simulink model "Target_Control_System"  (R2021b)
settings: Solver=FixedStepDiscrete  StartTime=0.0  StopTime=5  RelTol=1e-3
PreLoadFcn:
  | RTWConfigurationCB('preloadfcn', bdroot);
PostLoadFcn:
  | load('configuration/data_struct.mat');
  | load('configuration/fluxMaps_propMotor.mat');
  | load('configuration/parameterInit_PROP.mat');
  | load('configuration/parameterInit_PUMP.mat');
  | load('configuration/parameterInit_PITCH.mat');
  | load('configuration/parameterInit_TILT.mat');
  | %load('configuration/base_workspace_signal_definition.mat');
  | %load('resolvedatastores_to_baseworkspace_for_faster_simulation.mat');
model workspace (MAT data in the model file):
  SIMULATION_OPTIONS : Simulink.Parameter (value not decoded)
  TARGET_CODE_GEN : Simulink.Parameter (value not decoded)
  TCS_SAMPLE_FREQ_HZ : Simulink.Parameter (value not decoded)
symbols that are objects in the model workspace (value not decoded): TARGET_CODE_GEN, TCS_SAMPLE_FREQ_HZ
undefined symbols (not defined in the file): A_DQ_REF_LPF_INIT__PITCH, A_DQ_REF_LPF_INIT__PROP, A_DQ_REF_LPF_INIT__PUMP, A_DQ_REF_LPF_INIT__TILT, A_OBSERVER_CONFIDENCE_INIT__PITCH, A_OBSERVER_CONFIDENCE_INIT__PROP, A_OBSERVER_CONFIDENCE_INIT__PUMP, A_OBSERVER_CONFIDENCE_INIT__TILT, ACTUATOR_MAX_ANGLE_TRIP__PITCH, ACTUATOR_MIN_ANGLE_TRIP__PITCH, ACTUATOR_POS_SENSOR_INV_DIRECTION__PITCH, ACTUATOR_POS_SENSOR_INV_DIRECTION__TILT, ACTUATOR_POS_SENSOR_OFFSET__PITCH, ACTUATOR_POS_SENSOR_OFFSET__TILT, ADC_scaler1_baseaddr_TILT, ADC_SCALER_FLOAT_TO_FIXPOINT_EXPANSION, ANGLE_ELEC_FROM_SENSOR_OFFSET_INIT__PITCH, ANGLE_ELEC_FROM_SENSOR_OFFSET_INIT__PROP, ANGLE_ELEC_FROM_SENSOR_OFFSET_INIT__PUMP, ANGLE_ELEC_FROM_SENSOR_OFFSET_INIT__TILT, AUTO_CLEAR_FAULTS_ENABLED__PITCH, AUTO_CLEAR_FAULTS_ENABLED__PROP, AUTO_CLEAR_FAULTS_ENABLED__PUMP, AUTO_CLEAR_FAULTS_ENABLED__TILT, AUTO_CLEAR_FAULTS_WAIT_TICKS__PITCH, AUTO_CLEAR_FAULTS_WAIT_TICKS__PROP, AUTO_CLEAR_FAULTS_WAIT_TICKS__PUMP, AUTO_CLEAR_FAULTS_WAIT_TICKS__TILT, AUTO_I_ZERO_IDLE_TICKS__PITCH, AUTO_I_ZERO_IDLE_TICKS__PROP, AUTO_I_ZERO_IDLE_TICKS__PUMP, AUTO_I_ZERO_IDLE_TICKS__TILT, AUTO_I_ZERO_OFFSET_IDC_THRESHOLD__PITCH, AUTO_I_ZERO_OFFSET_IDC_THRESHOLD__PROP, AUTO_I_ZERO_OFFSET_IDC_THRESHOLD__PUMP, AUTO_I_ZERO_OFFSET_IDC_THRESHOLD__TILT, AUTO_I_ZERO_OFFSET_IPH_THRESHOLD__PITCH, AUTO_I_ZERO_OFFSET_IPH_THRESHOLD__PROP, AUTO_I_ZERO_OFFSET_IPH_THRESHOLD__PUMP, AUTO_I_ZERO_OFFSET_IPH_THRESHOLD__TILT, AUTO_SENSORLESS_SWITCHOVER_DISABLE_OMEGA, AUTO_SENSORLESS_SWITCHOVER_ENABLE_OMEGA, AUTO_SENSORLESS_SWITCHOVER_MIN_CONFIDENCE, AUXILIARY_PROTECTION_UNIT_BASEADDR__TILT, blanking_max_error_omega_INIT_PITCH, blanking_max_error_omega_INIT_TILT, blanking_max_error_position_INIT_PITCH, blanking_max_error_position_INIT_TILT, BRUTE_START_I_Q_REF_RAMP_SPEED__PITCH, BRUTE_START_I_Q_REF_RAMP_SPEED__PROP, BRUTE_START_I_Q_REF_RAMP_SPEED__PUMP, BRUTE_START_I_Q_REF_RAMP_SPEED__TILT, CONTROL_LOOP_DT_INIT__PITCH, CONTROL_LOOP_DT_INIT__PROP, CONTROL_LOOP_DT_INIT__PUMP, CONTROL_LOOP_DT_INIT__TILT, CORRECTION_FILTER_SCALE__PITCH, CORRECTION_FILTER_SCALE__PROP, CORRECTION_FILTER_SCALE__PUMP, CORRECTION_FILTER_SCALE__TILT ... (+458)
libraries: simulink x178, Reusables_Lib x24
(part 29 of 47)

== system Target_Control_System/Target_Control_System/MainLoop/pumpMotor_mainLoop/motorTaskMainFastStep(&oPump)/Control Loops - Pump/Dynamic Current Limiting Pump ==
  Enable : EnablePort
  Abs : Abs
  Add : Sum  Inputs=+-
  Add1 : Sum
  Add2 : Sum  Inputs=-+
  Data Store Read : DataStoreRead  DataStoreName=oPump  DataStoreElements=oPump.oMot_.oIn_.fIPhaseMagnitude_  IndexOptions=Index vector (dialog)  Indices=1  OutputSizes=1
  Data Store Read1 : DataStoreRead  DataStoreName=oPump  DataStoreElements=oPump.oMot_.oParam_.fIqSetpointMax_  IndexOptions=Index vector (dialog)  Indices=1  OutputSizes=1
  Data Store Read10 : DataStoreRead  DataStoreName=oPump  DataStoreElements=oPump.oMot_.oParam_.fDynILimIntegratorLeakageFactor_  IndexOptions=Index vector (dialog)  Indices=1  OutputSizes=1
  Data Store Read2 : DataStoreRead  DataStoreName=oPump  DataStoreElements=oPump.oMot_.oState_.fDynILimIntegrator_  IndexOptions=Index vector (dialog)  Indices=1  OutputSizes=1
  Data Store Read3 : DataStoreRead  DataStoreName=oPump  DataStoreElements=oPump.oMot_.oParam_.fDynILimDynamicMax_  IndexOptions=Index vector (dialog)  Indices=1  OutputSizes=1
  Data Store Read4 : DataStoreRead  DataStoreName=oPump  DataStoreElements=oPump.oMot_.oParam_.fTorqueAuthorityFraction_  IndexOptions=Index vector (dialog)  Indices=1  OutputSizes=1
  Data Store Read5 : DataStoreRead  DataStoreName=oPump  DataStoreElements=oPump.oMot_.oParam_.fDynILimKnockdownFactor_  IndexOptions=Index vector (dialog)  Indices=1  OutputSizes=1
  Data Store Read6 : DataStoreRead  DataStoreName=oPump  DataStoreElements=oPump.oMot_.oState_.fIqRefBeforeRamp_  IndexOptions=Index vector (dialog)  Indices=1  OutputSizes=1
  Data Store Read7 : DataStoreRead  DataStoreName=oPump  DataStoreElements=oPump.oMot_.oParam_.fDynILimDynamicMax_  IndexOptions=Index vector (dialog)  Indices=1  OutputSizes=1
  Data Store Write : DataStoreWrite  DataStoreName=oPump  DataStoreElements=oPump.oMot_.oState_.fDynILimIntegrator_  IndexOptions=Index vector (dialog)  Indices=1  OutputSizes=1
  Data Store Write1 : DataStoreWrite  DataStoreName=oPump  DataStoreElements=oPump.oMot_.oState_.fDynILimActualLimit_  IndexOptions=Index vector (dialog)  Indices=1  OutputSizes=1
  Data Store Write3 : DataStoreWrite  DataStoreName=oPump  DataStoreElements=oPump.oMot_.oParam_.oPid2DataRpmCtrl_.oParameter_.fOutMax_  IndexOptions=Index vector (dialog)  Indices=1  OutputSizes=1
  Data Store Write4 : DataStoreWrite  DataStoreName=oPump  DataStoreElements=oPump.oMot_.oParam_.oPid2DataRpmCtrl_.oParameter_.fOutMin_  IndexOptions=Index vector (dialog)  Indices=1  OutputSizes=1
  Data Store Write5 : DataStoreWrite  DataStoreName=oPump  DataStoreElements=oPump.oMot_.oParam_.oPid2DataRpmCtrl_.oParameter_.fIntMin_  IndexOptions=Index vector (dialog)  Indices=1  OutputSizes=1
  Data Store Write6 : DataStoreWrite  DataStoreName=oPump  DataStoreElements=oPump.oMot_.oParam_.oPid2DataRpmCtrl_.oParameter_.fIntMax_  IndexOptions=Index vector (dialog)  Indices=1  OutputSizes=1
  Divide{,1..3} (4 alike) : Product  Inputs=**
  Gain : Gain  Gain=-1
  Gain1 : Gain  Gain=-1
  Gain2 : Gain  Gain=-1
  Max : MinMax  Function=max  Inputs=2
  Max1 : MinMax  Function=max  Inputs=2
  Min : MinMax  Inputs=2
  Switch : Switch  Criteria=u2 > Threshold
  oRampDataIqRef_.fSetpoint : Outport
  wires:
  Gain2/1 -> Data Store Write4/1
  Data Store Read7/1 -> Gain2/1, Data Store Write3/1
  Gain1/1 -> Data Store Write5/1
  Max1/1 -> oRampDataIqRef_.fSetpoint/1
  Gain/1 -> Max1/1
  Min/1 -> Max1/2
  Data Store Read6/1 -> Min/2
  Max/1 -> Min/1, Data Store Write1/1, Gain1/1, Data Store Write6/1, Gain/1
  Add2/1 -> Max/1
  Divide2/1 -> Add2/2
  Divide3/1 -> Add2/1
  Data Store Read5/1 -> Divide3/2
  Data Store Read4/1 -> Divide2/2
  Data Store Read3/1 -> Divide2/1
  Divide1/1 -> Switch/3
  Data Store Read10/1 -> Divide1/2
  Data Store Read2/1 -> Add1/2, Divide1/1
  Divide/1 -> Add1/1
  Switch/1 -> Divide3/1, Data Store Write/1
  Add1/1 -> Switch/1
  Add/1 -> Switch/2, Divide/2, Divide/1  "fTemp"
  Abs/1 -> Add/1
  Data Store Read1/1 -> Add/2, Max/2
  Data Store Read/1 -> Abs/1

== system Target_Control_System/Target_Control_System/MainLoop/pumpMotor_mainLoop/motorTaskMainFastStep(&oPump)/Control Loops - Pump/Sim Options Prop Id Variant Subsystem ==
  note: 1) Add Subsystem or Model blocks as valid variant choices.
      | 2) You cannot connect blocks at this level. At simulation, connectivity is automatically
      | determined, based on the active variant and port name matching.
  Sim Options 0 Prop Id Subsystem : Subsystem  VariantControl=(default)
  Sim Options 1 Prop Id Subsystem : Subsystem  VariantControl=SIMULATION_OPTIONS == 1 && TARGET_CODE_GEN ~= 1
  Out1 : Outport

== system Target_Control_System/Target_Control_System/MainLoop/pumpMotor_mainLoop/motorTaskMainFastStep(&oPump)/Control Loops - Pump/Sim Options Pump Iq Variant Subsystem ==
  note: 1) Add Subsystem or Model blocks as valid variant choices.
      | 2) You cannot connect blocks at this level. At simulation, connectivity is automatically
      | determined, based on the active variant and port name matching.
  Sim Options 0 Pump Iq Subsystem : Subsystem  VariantControl=(default)
  Sim Options 1 Pump Iq Subsystem : Subsystem  VariantControl=SIMULATION_OPTIONS == 1 && TARGET_CODE_GEN ~= 1
  fSetpoint_ : Outport

== system Target_Control_System/Target_Control_System/MainLoop/pumpMotor_mainLoop/motorTaskMainFastStep(&oPump)/Control Loops - Pump/Sim Options Pump OmegaERef Variant Subsystem ==
  note: 1) Add Subsystem or Model blocks as valid variant choices.
      | 2) You cannot connect blocks at this level. At simulation, connectivity is automatically
      | determined, based on the active variant and port name matching.
  Sim Options 0 Pump OmegaE Subsystem : Subsystem  VariantControl=(default)
  Sim Options 1 Pump OmegaE Subsystem : Subsystem  VariantControl=SIMULATION_OPTIONS == 1 && TARGET_CODE_GEN ~= 1
  Out1 : Outport

== system Target_Control_System/Target_Control_System/MainLoop/pumpMotor_mainLoop/motorTaskMainFastStep(&oPump)/Control Loops - Pump/Subsystem ==
  note: // Drives without sensors use the PI type controller and the estimated speed
  note: // Drives with sensors use the PID2 controller and the sensor (derived or reported) speed
  note: // Drive states 245-255 are for resistance measurement
  In Bus Element : Inport  PortName=oRampDataOmegaERef_.fRampOut
  In Bus Element1 : Inport  PortName=oRampDataOmegaERef_.fRampOut
  Enable : EnablePort
  AND : Logic  AllPortsSameDT=off  OutDataTypeStr=boolean
  Constant : Constant  OutDataTypeStr=single  SampleTime=-1
  Constant1 : Constant  OutDataTypeStr=single  SampleTime=-1
  Constant2 : Constant  Value=245  OutDataTypeStr=uint32  SampleTime=-1
  Data Store Read2 : DataStoreRead  DataStoreName=oPump  DataStoreElements=oPump.oMot_.oIn_.fOmegaEObserverLpf2_  IndexOptions=Index vector (dialog)  Indices=1  OutputSizes=1
  Data Store Read4 : DataStoreRead  DataStoreName=oPump  DataStoreElements=oPump.oMot_.oParam_.oPid2DataRpmCtrl_.fState_  IndexOptions=Index vector (dialog)  Indices=1  OutputSizes=1
  Data Store Read5 : DataStoreRead  DataStoreName=oPump  DataStoreElements=oPump.oMot_.oParam_.uiTorqueMirroringActive_  IndexOptions=Index vector (dialog)  Indices=1  OutputSizes=1
  Data Store Read6 : DataStoreRead  DataStoreName=oPump  DataStoreElements=oPump.oMot_.oState_.uiDriveState_  IndexOptions=Index vector (dialog)  Indices=1  OutputSizes=1
  Data Store Read62 : DataStoreRead  DataStoreName=oPump  DataStoreElements=oPump.oIsr_.oParam_.iUseSensorAngle_  IndexOptions=Index vector (dialog)  Indices=1  OutputSizes=1
  Data Store Read7 : DataStoreRead  DataStoreName=oPump  DataStoreElements=oPump.oMot_.oState_.oPosSensor_.fOmegaEFromSensor_  IndexOptions=Index vector (dialog)  Indices=1  OutputSizes=1
  Data Store Write19 : DataStoreWrite  DataStoreName=oPump  DataStoreElements=oPump.oMot_.oState_.fIqRefBeforeRamp_  IndexOptions=Index vector (dialog)  Indices=1  OutputSizes=1
  Data Store Write5 : DataStoreWrite  DataStoreName=oPump  DataStoreElements=oPump.oMot_.oState_.fIqRefFromSpeedController_  IndexOptions=Index vector (dialog)  Indices=1  OutputSizes=1
  Less Than : RelationalOperator  Operator=<  OutDataTypeStr=boolean  RndMeth=Simplest
  NOT : Logic  Operator=NOT  AllPortsSameDT=off  OutDataTypeStr=boolean
  NOT1 : Logic  Operator=NOT  AllPortsSameDT=off  OutDataTypeStr=boolean
  Set Iq Ref Pump : Subsystem  TreatAsAtomicUnit=on
  Switch : Switch  Criteria=u2 > Threshold
  piControllerStep(&oPiDataRpm_) : Subsystem
  pid2ControllerStep(&oPid2DataRpmCtrl_) : Subsystem
  wires:
  Set Iq Ref Pump/1(fIqRefBeforeRamp) -> Data Store Write19/1
  AND/1 -> Set Iq Ref Pump/Enable
  Less Than/1 -> AND/2
  NOT1/1 -> AND/1
  Data Store Read5/1 -> NOT1/1
  Data Store Read6/1 -> Less Than/1
  Constant2/1 -> Less Than/2
  Switch/1 -> Data Store Write5/1, Set Iq Ref Pump/1(fIqRefFromSpeedController)
  pid2ControllerStep(&oPid2DataRpmCtrl_)/1(fOutput) -> Switch/1
  Data Store Read7/1 -> pid2ControllerStep(&oPid2DataRpmCtrl_)/2(fActual)
  Data Store Read4/1 -> pid2ControllerStep(&oPid2DataRpmCtrl_)/1(fState)
  Constant1/1 -> pid2ControllerStep(&oPid2DataRpmCtrl_)/4(fActualDdt)
  In Bus Element/1 -> pid2ControllerStep(&oPid2DataRpmCtrl_)/3(fTarget)
  Data Store Read2/1 -> piControllerStep(&oPiDataRpm_)/1(fActual)
  piControllerStep(&oPiDataRpm_)/1(fOutput) -> Switch/3
  In Bus Element1/1 -> piControllerStep(&oPiDataRpm_)/2(fTarget)
  Constant/1 -> piControllerStep(&oPiDataRpm_)/3(fScale)
  Data Store Read62/1 -> Switch/2, pid2ControllerStep(&oPid2DataRpmCtrl_)/Enable, NOT/1
  NOT/1 -> piControllerStep(&oPiDataRpm_)/Enable

== system Target_Control_System/Target_Control_System/MainLoop/pumpMotor_mainLoop/motorTaskMainFastStep(&oPump)/Control Loops - Pump/Subsystem2 ==
  Enable : EnablePort
  Data Store Read2 : DataStoreRead  DataStoreName=oPump  DataStoreElements=oPump.oMot_.oIn_.fUdRef_  IndexOptions=Index vector (dialog)  Indices=1  OutputSizes=1
  Data Store Read3 : DataStoreRead  DataStoreName=oPump  DataStoreElements=oPump.oMot_.oIn_.fUqRef_  IndexOptions=Index vector (dialog)  Indices=1  OutputSizes=1
  Data Store Read5 : DataStoreRead  DataStoreName=oPump  DataStoreElements=oPump.oMot_.oState_.fFluxWeakeningState_  IndexOptions=Index vector (dialog)  Indices=1  OutputSizes=1
  Data Store Read6 : DataStoreRead  DataStoreName=oPump  DataStoreElements=oPump.oMot_.oParam_.fFluxWeakeningModulationTarget_  IndexOptions=Index vector (dialog)  Indices=1  OutputSizes=1
  Data Store Read69 : DataStoreRead  DataStoreName=oPump  DataStoreElements=oPump.oMot_.oParam_.fFluxWeakeningDownRamp_  IndexOptions=Index vector (dialog)  Indices=1  OutputSizes=1
  Data Store Read94 : DataStoreRead  DataStoreName=oPump  DataStoreElements=oPump.oMot_.oState_.fFluxWeakeningState_  IndexOptions=Index vector (dialog)  Indices=1  OutputSizes=1
  Data Store Read95 : DataStoreRead  DataStoreName=oPump  DataStoreElements=oPump.oMot_.oParam_.fIntControlLoopDt_  IndexOptions=Index vector (dialog)  Indices=1  OutputSizes=1
  Data Store Read96 : DataStoreRead  DataStoreName=oPump  DataStoreElements=oPump.oMot_.oParam_.fIntControlLoopDt_  IndexOptions=Index vector (dialog)  Indices=1  OutputSizes=1
  Equal13 : RelationalOperator  Operator=<  OutDataTypeStr=boolean  RndMeth=Simplest
  Mux : Mux  Inputs=2
  NOT1 : Logic  Operator=NOT  AllPortsSameDT=off  OutDataTypeStr=boolean
  Square Sum : Fcn  Expr=u(1)*u(1)+u(2)*u(2)
  Subsystem : Subsystem
  Subsystem1 : Subsystem
  Switch1 : Switch  Criteria=u2 > Threshold  Threshold=0.5
  Out1 : Outport
  wires:
  Subsystem1/1(Out1) -> Switch1/1
  NOT1/1 -> Subsystem/Enable
  Data Store Read94/1 -> Subsystem/3(fFluxWeakeningState_)
  Subsystem/1(Out1) -> Switch1/3
  Mux/1 -> Square Sum/1
  Data Store Read95/1 -> Subsystem/4(fIntControlLoopDt_)
  Data Store Read6/1 -> Equal13/2, Subsystem/1(fFluxWeakeningModulationTarget_)  "fFluxWeakeningModulationTarget_"
  Square Sum/1 -> Subsystem/2(fModulationIndexSquared), Equal13/1  "fModulationIndexSquared_"
  Data Store Read3/1 -> Mux/2
  Equal13/1 -> Subsystem1/Enable, NOT1/1, Switch1/2
  Data Store Read96/1 -> Subsystem1/2(fIntControlLoopDt_)
  Switch1/1 -> Out1/1
  Data Store Read2/1 -> Mux/1
  Data Store Read69/1 -> Subsystem1/1(fFluxWeakeningDownRamp_)
  Data Store Read5/1 -> Subsystem1/3(fFluxWeakeningState_)

== system Target_Control_System/Target_Control_System/MainLoop/pumpMotor_mainLoop/motorTaskMainFastStep(&oPump)/Control Loops - Pump/rampStep_oRampDataIqRef_ ==
  note: U(k)
  note: Y(k)
  fSetpoint_ : Inport
  fUpslope_ : Inport  Port=2
  fDDownslope_ : Inport  Port=3
  fTimestepS_ : Inport  Port=4
  fRampOut_z : Inport  Port=5
  Difference Inputs1 : Sum  Description=Add in CPU  DisableCoverage=on  Inputs=+-  OutDataTypeStr=Inherit: Inherit via back propagation
  Difference Inputs2 : Sum  Description=Add in CPU  OutDataTypeStr=Inherit: Inherit via back propagation
  Difference Inputs3 : Sum  Description=Add in CPU  DisableCoverage=on  Inputs=+-  OutDataTypeStr=Inherit: Inherit via back propagation
  Gain : Gain  Gain=-1
  Saturation Dynamic : simulink/Discontinuities/Saturation Dynamic  OutMin=[]  OutMax=[]  OutDataTypeStr=Inherit: Same as second input  OutDataType=fixdt(1, 16)  OutScaling=2^-10  DoSatur=off
  delta fall limit : Product  DisableCoverage=on  Inputs=**  OutDataTypeStr=Inherit: Inherit via back propagation  SaturateOnIntegerOverflow=on
  delta fall limit1 : Product  DisableCoverage=on  Inputs=*/  OutDataTypeStr=Inherit: Inherit via back propagation  SaturateOnIntegerOverflow=on
  delta rise limit : Product  DisableCoverage=on  Inputs=**  OutDataTypeStr=Inherit: Inherit via back propagation  SaturateOnIntegerOverflow=on
  fRampOut_ : Outport  InitialOutput=0
  fRampOutDdt_ : Outport  Port=2  InitialOutput=0
  wires:
  fRampOut_z/1 -> Difference Inputs1/2, Difference Inputs2/2, Difference Inputs3/2
  Difference Inputs1/1 -> Saturation Dynamic/2  "( U(k) - Y(k-1) )"
  fDDownslope_/1 -> Gain/1
  delta rise limit/1 -> Saturation Dynamic/1
  fSetpoint_/1 -> Difference Inputs1/1
  delta fall limit/1 -> Saturation Dynamic/3
  fUpslope_/1 -> delta rise limit/1
  Difference Inputs2/1 -> Difference Inputs3/1, fRampOut_/1
  Saturation Dynamic/1 -> Difference Inputs2/1
  fTimestepS_/1 -> delta fall limit1/2, delta fall limit/2, delta rise limit/2
  Difference Inputs3/1 -> delta fall limit1/1  "( Y(k) - Y(k-1) )"
  delta fall limit1/1 -> fRampOutDdt_/1
  Gain/1 -> delta fall limit/1

== system Target_Control_System/Target_Control_System/MainLoop/pumpMotor_mainLoop/motorTaskMainFastStep(&oPump)/Correction Constants for Observer and Control - Pump/Variant Subsystem ==
  note: 1) Add Subsystem or Model blocks as valid variant choices.
      | 2) You cannot connect blocks at this level. At simulation, connectivity is automatically
      | determined, based on the active variant and port name matching.
  In1 : Inport
  Simulation Subsystem IIR Voltage Filter Freq : Subsystem  TreatAsAtomicUnit=on  VariantControl=TARGET_CODE_GEN == 0
  Target Code Gen Subsystem IIR Voltage Filter Freq : Subsystem  TreatAsAtomicUnit=on  VariantControl="TARGET_CODE_GEN  == 1"
  Out1 : Outport

== system Target_Control_System/Target_Control_System/MainLoop/pumpMotor_mainLoop/motorTaskMainFastStep(&oPump)/Observer Confidence - Pump/IIR ==
  In : Inport
  1-K : Inport  Port=2
  K : Inport  Port=3
  Product : Product  OutDataTypeStr=single  RndMeth=Zero
  Product1 : Product  RndMeth=Zero
  Sum : Sum  Inputs=|++  OutDataTypeStr=single
  Unit Delay : UnitDelay  SampleTime=-1  HasFrameUpgradeWarning=on
  Out : Outport
  wires:
  Sum/1 -> Unit Delay/1, Out/1
  Unit Delay/1 -> Product/1
  K/1 -> Product1/2
  1-K/1 -> Product/2
  Product/1 -> Sum/1
  Product1/1 -> Sum/2
  In/1 -> Product1/1

== system Target_Control_System/Target_Control_System/MainLoop/pumpMotor_mainLoop/motorTaskMainFastStep(&oPump)/PWM for Simulation/Subsystem ==
  Enable : EnablePort
  Bus Creator1 : BusCreator  Inputs=3
  Data Store Read7 : DataStoreRead  DataStoreName=oPump  DataStoreElements=oPump.oIsr_.oOut_.uiPwmDutyTicksA_  IndexOptions=Index vector (dialog)  Indices=1  OutputSizes=1
  Data Store Read8 : DataStoreRead  DataStoreName=oPump  DataStoreElements=oPump.oIsr_.oOut_.uiPwmDutyTicksB_  IndexOptions=Index vector (dialog)  Indices=1  OutputSizes=1
  Data Store Read9 : DataStoreRead  DataStoreName=oPump  DataStoreElements=oPump.oIsr_.oOut_.uiPwmDutyTicksC_  IndexOptions=Index vector (dialog)  Indices=1  OutputSizes=1
  pumpMotor_PWMticks : Outport
  wires:
  Data Store Read8/1 -> Bus Creator1/2  "Bticks"
  Bus Creator1/1 -> pumpMotor_PWMticks/1
  Data Store Read9/1 -> Bus Creator1/3  "Cticks"
  Data Store Read7/1 -> Bus Creator1/1  "Aticks"

== system Target_Control_System/Target_Control_System/MainLoop/pumpMotor_mainLoop/motorTaskMainFastStep(&oPump)/PWM for Simulation/Subsystem1 ==
  Enable : EnablePort
  Data Store Read6 : DataStoreRead  DataStoreName=oPump  DataStoreElements=oPump.oMot_.oOut_.uiPwmRequestFromMain_  IndexOptions=Index vector (dialog)  Indices=1  OutputSizes=1
  Scope : Scope
  Subsystem : Subsystem
  pumpMotor_PWMticks : Outport
  wires:
  Data Store Read6/1 -> Subsystem/Enable, Scope/1
  Subsystem/1(pumpMotor_PWMticks) -> pumpMotor_PWMticks/1

== system Target_Control_System/Target_Control_System/MainLoop/pumpMotor_mainLoop/motorTaskMainFastStep(&oPump)/Variant Subsystem/Target_Code_Gen_0 ==
  Function-Call Generator : simulink/Ports & Subsystems/Function-Call Generator  sample_time=-1  numberOfIterations=1  DisallowWideOutput=off
  Output : Outport
  wires:
  Function-Call Generator/1 -> Output/1

== system Target_Control_System/Target_Control_System/MainLoop/pumpMotor_mainLoop/motorTaskMainFastStep(&oPump)/Variant Subsystem/Target_Code_Gen_1 ==
  Data Store Read16 : DataStoreRead  DataStoreName=oPump  DataStoreElements=oPump.oMot_.oIn_.uiDataFromIsrToMainUpdated_  IndexOptions=Index vector (dialog)  Indices=1  OutputSizes=1
  Triggered Subsystem : Subsystem  TreatAsAtomicUnit=on
  Output : Outport
  wires:
  Triggered Subsystem/1(Output) -> Output/1
  Data Store Read16/1 -> Triggered Subsystem/Trigger

== system Target_Control_System/Target_Control_System/MainLoop/tiltMotor_mainLoop/Decimation gate for 10 Hz Tilt/Function-Call Subsystem/Dynamic_current_limiting ==
  Constant : Constant  Value=0  OutDataTypeStr=single  SampleTime=-1
  Data Store Read2 : DataStoreRead  DataStoreName=oTilt  DataStoreElements=oTilt.oMot_.oParam_.fDynILimIntegratorLeakageFactor_  IndexOptions=Index vector (dialog)  Indices=1  OutputSizes=1
  Enabled Subsystem : Subsystem  TreatAsAtomicUnit=on
  GreaterThan : RelationalOperator  Operator=>  OutDataTypeStr=boolean  RndMeth=Simplest
  wires:
  GreaterThan/1 -> Enabled Subsystem/Enable
  Data Store Read2/1 -> GreaterThan/1
  Constant/1 -> GreaterThan/2

== system Target_Control_System/Target_Control_System/MainLoop/tiltMotor_mainLoop/Decimation gate for 200 Hz Tilt/motorTaskMainDecimationAStep(&oTilt)/Check zero current if inverter off ==
  function : TriggerPort  TriggerType=function-call  VariantControl=Variant
  AND : Logic  Inputs=3  AllPortsSameDT=off  OutDataTypeStr=boolean
  Constant : Constant  Value=200  OutDataTypeStr=uint32  SampleTime=-1
  Constant1 : Constant  Value=99  OutDataTypeStr=uint32  SampleTime=-1
  Constant2 : Constant  Value=0  OutDataTypeStr=uint32  SampleTime=-1
  Data Store Read1 : DataStoreRead  DataStoreName=oTilt  DataStoreElements=oTilt.oMot_.oState_.uiDriveState_  IndexOptions=Index vector (dialog)  Indices=1  OutputSizes=1
  Data Store Read2 : DataStoreRead  DataStoreName=oTilt  DataStoreElements=oTilt.oMot_.oState_.uiCurrentOffsetNullingPerformed_  IndexOptions=Index vector (dialog)  Indices=1  OutputSizes=1
  Enabled Subsystem : Subsystem  TreatAsAtomicUnit=on
  GreaterThan : RelationalOperator  Operator=>  OutDataTypeStr=boolean  RndMeth=Simplest
  GreaterThan1 : RelationalOperator  Operator=>  OutDataTypeStr=boolean  RndMeth=Simplest
  Less Than : RelationalOperator  Operator=<  OutDataTypeStr=boolean  RndMeth=Simplest
  wires:
  AND/1 -> Enabled Subsystem/Enable
  GreaterThan1/1 -> AND/3
  Constant2/1 -> GreaterThan1/2
  Data Store Read2/1 -> GreaterThan1/1
  Less Than/1 -> AND/2
  GreaterThan/1 -> AND/1
  Constant1/1 -> GreaterThan/2
  Constant/1 -> Less Than/2
  Data Store Read1/1 -> GreaterThan/1, Less Than/1

== system Target_Control_System/Target_Control_System/MainLoop/tiltMotor_mainLoop/Decimation gate for 200 Hz Tilt/motorTaskMainDecimationAStep(&oTilt)/Current control inactive ==
  function : TriggerPort  TriggerType=function-call  VariantControl=Variant
  Constant : Constant  Value=0  OutDataTypeStr=uint32  SampleTime=-1
  Data Store Read : DataStoreRead  DataStoreName=oTilt  DataStoreElements=oTilt.oMot_.oOut_.uiCurrentControllerActive_  IndexOptions=Index vector (dialog)  Indices=1  OutputSizes=1
  Enabled Subsystem : Subsystem  TreatAsAtomicUnit=on
  GreaterThan : RelationalOperator  Operator=>  OutDataTypeStr=boolean  RndMeth=Simplest
  NOT : Logic  Operator=NOT  IconShape=distinctive  AllPortsSameDT=off  OutDataTypeStr=boolean
  wires:
  NOT/1 -> Enabled Subsystem/Enable
  GreaterThan/1 -> NOT/1
  Constant/1 -> GreaterThan/2
  Data Store Read/1 -> GreaterThan/1

== system Target_Control_System/Target_Control_System/MainLoop/tiltMotor_mainLoop/Decimation gate for 200 Hz Tilt/motorTaskMainDecimationAStep(&oTilt)/Current offset nulling ==
  note: Try to perform current sensor offset nulling at least once as soon as possible:
      | (Subsequent nulling steps are performed only once the drive has been idle for a while)
  function : TriggerPort  TriggerType=function-call  VariantControl=Variant
  Constant2 : Constant  Value=0  OutDataTypeStr=uint32  SampleTime=-1
  Data Store Read2 : DataStoreRead  DataStoreName=oTilt  DataStoreElements=oTilt.oMot_.oState_.uiCurrentOffsetNullingPerformed_  IndexOptions=Index vector (dialog)  Indices=1  OutputSizes=1
  GreaterThan1 : RelationalOperator  Operator=>  OutDataTypeStr=boolean  RndMeth=Simplest
  NOT : Logic  Operator=NOT  IconShape=distinctive  AllPortsSameDT=off  OutDataTypeStr=boolean
  initiateOffsetNulling(&oTilt) : Subsystem  TreatAsAtomicUnit=on
  wires:
  NOT/1 -> initiateOffsetNulling(&oTilt)/Enable
  GreaterThan1/1 -> NOT/1
  Constant2/1 -> GreaterThan1/2
  Data Store Read2/1 -> GreaterThan1/1

== system Target_Control_System/Target_Control_System/MainLoop/tiltMotor_mainLoop/Decimation gate for 200 Hz Tilt/motorTaskMainDecimationAStep(&oTilt)/DClink_overCurrentProtection ==
  function : TriggerPort  TriggerType=function-call  VariantControl=Variant
  Chart : Stateflow chart  TreatAsAtomicUnit=on

== system Target_Control_System/Target_Control_System/MainLoop/tiltMotor_mainLoop/Decimation gate for 200 Hz Tilt/motorTaskMainDecimationAStep(&oTilt)/Forced current injection for broken input sensors ==
  function : TriggerPort  TriggerType=function-call  VariantControl=Variant
  Constant : Constant  Value=226  OutDataTypeStr=uint32  SampleTime=-1
  Constant1 : Constant  Value=227  OutDataTypeStr=uint32  SampleTime=-1
  Constant2 : Constant  Value=228  OutDataTypeStr=uint32  SampleTime=-1
  Data Store Read : DataStoreRead  DataStoreName=oTilt  DataStoreElements=oTilt.oMot_.oState_.uiDriveState_  IndexOptions=Index vector (dialog)  Indices=1  OutputSizes=1
  Enabled Subsystem : Subsystem  TreatAsAtomicUnit=on
  Equal : RelationalOperator  Operator===  OutDataTypeStr=boolean  RndMeth=Simplest
  Equal1 : RelationalOperator  Operator===  OutDataTypeStr=boolean  RndMeth=Simplest
  Equal2 : RelationalOperator  Operator===  OutDataTypeStr=boolean  RndMeth=Simplest
  OR : Logic  Operator=OR  Inputs=3  AllPortsSameDT=off  OutDataTypeStr=boolean
  wires:
  OR/1 -> Enabled Subsystem/Enable
  Equal2/1 -> OR/3
  Equal/1 -> OR/1
  Equal1/1 -> OR/2
  Constant2/1 -> Equal2/2
  Constant1/1 -> Equal1/2
  Constant/1 -> Equal/2
  Data Store Read/1 -> Equal/1, Equal1/1, Equal2/1

== system Target_Control_System/Target_Control_System/MainLoop/tiltMotor_mainLoop/Decimation gate for 200 Hz Tilt/motorTaskMainDecimationAStep(&oTilt)/Idle controller ==
  function : TriggerPort  TriggerType=function-call  VariantControl=Variant
  Constant : Constant  Value=211  OutDataTypeStr=uint32  SampleTime=-1
  Constant1 : Constant  Value=212  OutDataTypeStr=uint32  SampleTime=-1
  Data Store Read : DataStoreRead  DataStoreName=oTilt  DataStoreElements=oTilt.oMot_.oState_.uiDriveState_  IndexOptions=Index vector (dialog)  Indices=1  OutputSizes=1
  Equal : RelationalOperator  Operator===  OutDataTypeStr=boolean  RndMeth=Simplest
  Equal1 : RelationalOperator  Operator===  OutDataTypeStr=boolean  RndMeth=Simplest
  Forced angle : Subsystem  TreatAsAtomicUnit=on
  NOT : Logic  Operator=NOT  IconShape=distinctive  AllPortsSameDT=off  OutDataTypeStr=boolean
  Not forced angle : Subsystem  TreatAsAtomicUnit=on
  OR : Logic  Operator=OR  AllPortsSameDT=off  OutDataTypeStr=boolean
  wires:
  NOT/1 -> Not forced angle/Enable
  OR/1 -> NOT/1, Forced angle/Enable
  Equal1/1 -> OR/2
  Equal/1 -> OR/1
  Constant1/1 -> Equal1/2
  Data Store Read/1 -> Equal/1, Equal1/1
  Constant/1 -> Equal/2

== system Target_Control_System/Target_Control_System/MainLoop/tiltMotor_mainLoop/Decimation gate for 200 Hz Tilt/motorTaskMainDecimationAStep(&oTilt)/Position control checks ==
  function : TriggerPort  TriggerType=function-call  VariantControl=Variant
  Constant : Constant  Value=0  OutDataTypeStr=int32  SampleTime=-1
  Data Store Read : DataStoreRead  DataStoreName=oTilt  DataStoreElements=oTilt.oMot_.oState_.oPosSensor_.iPosControlEnabled_  IndexOptions=Index vector (dialog)  Indices=1  OutputSizes=1
  GreaterThan : RelationalOperator  Operator=>  OutDataTypeStr=boolean  RndMeth=Simplest
  NOT : Logic  Operator=NOT  IconShape=distinctive  AllPortsSameDT=off  OutDataTypeStr=boolean
  NOT position control mode : Subsystem  TreatAsAtomicUnit=on
  Position control mode : Subsystem  TreatAsAtomicUnit=on
  wires:
  NOT/1 -> NOT position control mode/Enable
  Constant/1 -> GreaterThan/2
  Data Store Read/1 -> GreaterThan/1
  GreaterThan/1 -> Position control mode/Enable, NOT/1

== system Target_Control_System/Target_Control_System/MainLoop/tiltMotor_mainLoop/Decimation gate for 5000 Hz Tilt/motorTaskProcessExternalSetpoints(&oTilt)/hot_standby ==
  hot_standby : TriggerPort  TriggerType=function-call  VariantControl=Variant
  AND5 : Logic  Operator=OR  AllPortsSameDT=off  OutDataTypeStr=boolean
  Data Store Read85 : DataStoreRead  DataStoreName=oTilt  DataStoreElements=oTilt.oMot_.oState_.uiDriveState_  IndexOptions=Index vector (dialog)  Indices=1  OutputSizes=1
  Equal1 : RelationalOperator  Operator===  OutDataTypeStr=boolean  RndMeth=Simplest
  Equal13 : RelationalOperator  Operator===  OutDataTypeStr=boolean  RndMeth=Simplest
  Subsystem : Subsystem
  const1 : Constant  Value=235  OutDataTypeStr=uint32  SampleTime=-1
  const2 : Constant  Value=236  OutDataTypeStr=uint32  SampleTime=-1
  wires:
  const2/1 -> Equal1/2
  const1/1 -> Equal13/2
  Data Store Read85/1 -> Equal13/1, Equal1/1
  Equal1/1 -> AND5/2
  AND5/1 -> Subsystem/Enable
  Equal13/1 -> AND5/1

== system Target_Control_System/Target_Control_System/MainLoop/tiltMotor_mainLoop/Decimation gate for 5000 Hz Tilt/motorTaskProcessExternalSetpoints(&oTilt)/passive_holding_mode ==
  passive_holding_mode : TriggerPort  TriggerType=function-call  VariantControl=Variant
  AND5 : Logic  Operator=OR  Inputs=3  AllPortsSameDT=off  OutDataTypeStr=boolean
  Data Store Read85 : DataStoreRead  DataStoreName=oTilt  DataStoreElements=oTilt.oMot_.oState_.uiDriveState_  IndexOptions=Index vector (dialog)  Indices=1  OutputSizes=1
  Equal1 : RelationalOperator  Operator===  OutDataTypeStr=boolean  RndMeth=Simplest
  Equal13 : RelationalOperator  Operator===  OutDataTypeStr=boolean  RndMeth=Simplest
  Equal2 : RelationalOperator  Operator===  OutDataTypeStr=boolean  RndMeth=Simplest
  Subsystem : Subsystem
  const1 : Constant  Value=226  OutDataTypeStr=uint32  SampleTime=-1
  const2 : Constant  Value=227  OutDataTypeStr=uint32  SampleTime=-1
  const3 : Constant  Value=228  OutDataTypeStr=uint32  SampleTime=-1
  wires:
  const3/1 -> Equal2/2
  const2/1 -> Equal1/2
  const1/1 -> Equal13/2
  Data Store Read85/1 -> Equal13/1, Equal1/1, Equal2/1
  Equal1/1 -> AND5/2
  Equal2/1 -> AND5/3
  AND5/1 -> Subsystem/Enable
  Equal13/1 -> AND5/1

== system Target_Control_System/Target_Control_System/MainLoop/tiltMotor_mainLoop/Decimation gate for 5000 Hz Tilt/motorTaskProcessExternalSetpoints(&oTilt)/set_target ==
  note: // Position target
  note: // Speed target
  note: Iq current (that is, torque target)
  note: // Do Id
  note: // (Iq is controlled by the forced angle sequencer)
  note: // Forced angle start regime, ensure that Id is zero
  set_target : TriggerPort  TriggerType=function-call  VariantControl=Variant
  AND1 : Logic  AllPortsSameDT=off  OutDataTypeStr=boolean
  AND5 : Logic  Inputs=3  AllPortsSameDT=off  OutDataTypeStr=boolean
  Data Store Read85 : DataStoreRead  DataStoreName=oTilt  DataStoreElements=oTilt.oMot_.oState_.uiDriveState_  IndexOptions=Index vector (dialog)  Indices=1  OutputSizes=1
  Equal1 : RelationalOperator  OutDataTypeStr=boolean  RndMeth=Simplest
  Equal13 : RelationalOperator  Operator=~=  OutDataTypeStr=boolean  RndMeth=Simplest
  Equal14 : RelationalOperator  Operator=~=  OutDataTypeStr=boolean  RndMeth=Simplest
  Equal2 : RelationalOperator  Operator=<=  OutDataTypeStr=boolean  RndMeth=Simplest
  Id_target : Subsystem
  Id_zero_for_forced_angle : Subsystem
  Iq_target : Subsystem
  NOT : Logic  Operator=NOT  AllPortsSameDT=off  OutDataTypeStr=boolean
  NOT1 : Logic  Operator=NOT  AllPortsSameDT=off  OutDataTypeStr=boolean
  const1 : Constant  Value=245  OutDataTypeStr=uint32  SampleTime=-1
  const17 : Constant  Value=211  OutDataTypeStr=uint32  SampleTime=-1
  const18 : Constant  Value=212  OutDataTypeStr=uint32  SampleTime=-1
  const2 : Constant  Value=254  OutDataTypeStr=uint32  SampleTime=-1
  position_target : Subsystem
  speed_target : Subsystem
  wires:
  NOT1/1 -> Id_zero_for_forced_angle/Enable
  AND5/1 -> NOT1/1, position_target/Enable, Iq_target/Enable, Id_target/Enable, speed_target/Enable
  Equal13/1 -> AND5/1
  Equal1/1 -> AND1/1
  const18/1 -> Equal14/2
  Equal2/1 -> AND1/2
  AND1/1 -> NOT/1
  const17/1 -> Equal13/1
  Data Store Read85/1 -> Equal2/1, Equal1/1, Equal14/1, Equal13/2
  const2/1 -> Equal2/2
  NOT/1 -> AND5/3
  const1/1 -> Equal1/2
  Equal14/1 -> AND5/2

== system Target_Control_System/Target_Control_System/MainLoop/tiltMotor_mainLoop/mainTask_tilt/PWM for Simulation/Subsystem ==
  Enable : EnablePort
  Bus Creator1 : BusCreator  Inputs=3
  Data Store Read7 : DataStoreRead  DataStoreName=oTilt  DataStoreElements=oTilt.oIsr_.oOut_.uiPwmDutyTicksA_  IndexOptions=Index vector (dialog)  Indices=1  OutputSizes=1
  Data Store Read8 : DataStoreRead  DataStoreName=oTilt  DataStoreElements=oTilt.oIsr_.oOut_.uiPwmDutyTicksB_  IndexOptions=Index vector (dialog)  Indices=1  OutputSizes=1
  Data Store Read9 : DataStoreRead  DataStoreName=oTilt  DataStoreElements=oTilt.oIsr_.oOut_.uiPwmDutyTicksC_  IndexOptions=Index vector (dialog)  Indices=1  OutputSizes=1
  tiltMotor_PWMticks : Outport
  wires:
  Data Store Read8/1 -> Bus Creator1/2  "Bticks"
  Bus Creator1/1 -> tiltMotor_PWMticks/1
  Data Store Read9/1 -> Bus Creator1/3  "Cticks"
  Data Store Read7/1 -> Bus Creator1/1  "Aticks"

== system Target_Control_System/Target_Control_System/MainLoop/tiltMotor_mainLoop/mainTask_tilt/PWM for Simulation/Subsystem1 ==
  Enable : EnablePort
  Data Store Read6 : DataStoreRead  DataStoreName=oTilt  DataStoreElements=oTilt.oMot_.oOut_.uiPwmRequestFromMain_  IndexOptions=Index vector (dialog)  Indices=1  OutputSizes=1
  Scope : Scope
  Subsystem : Subsystem
  tiltMotor_PWMticks : Outport
  wires:
  Data Store Read6/1 -> Subsystem/Enable, Scope/1
  Subsystem/1(tiltMotor_PWMticks) -> tiltMotor_PWMticks/1

== system Target_Control_System/Target_Control_System/MainLoop/tiltMotor_mainLoop/mainTask_tilt/Variant Subsystem/Target_Code_Gen_0 ==
  Function-Call Generator : simulink/Ports & Subsystems/Function-Call Generator  sample_time=-1  numberOfIterations=1  DisallowWideOutput=off
  Out1 : Outport
  wires:
  Function-Call Generator/1 -> Out1/1

== system Target_Control_System/Target_Control_System/MainLoop/tiltMotor_mainLoop/mainTask_tilt/Variant Subsystem/Target_Code_Gen_1 ==
  Data Store Read4 : DataStoreRead  DataStoreName=oTilt  DataStoreElements=oTilt.oMot_.oIn_.uiDataFromIsrToMainUpdated_  IndexOptions=Index vector (dialog)  Indices=1  OutputSizes=1
  Triggered Subsystem : Subsystem  TreatAsAtomicUnit=on
  Out1 : Outport
  wires:
  Triggered Subsystem/1(Output) -> Out1/1
  Data Store Read4/1 -> Triggered Subsystem/Trigger

== system Target_Control_System/Target_Control_System/MainLoop/tiltMotor_mainLoop/mainTask_tilt/motorTaskMainFastStep(&oTilt)/Automatic switching to sensorless - Tilt ==
  autoSwitchToSensorless : TriggerPort  TriggerType=function-call  VariantControl=Variant
  Automatic switching to sensorless : Subsystem  TreatAsAtomicUnit=on
  Constant : Constant  Value=0  SampleTime=-1
  Data Store Read3 : DataStoreRead  DataStoreName=oTilt  DataStoreElements=oTilt.oMot_.oParam_.uiSensorlessSwitchoverMode_  IndexOptions=Index vector (dialog)  Indices=1  OutputSizes=1
  GreaterThan : RelationalOperator  Operator=>  OutDataTypeStr=boolean  RndMeth=Simplest
  wires:
  Constant/1 -> GreaterThan/2
  GreaterThan/1 -> Automatic switching to sensorless/Enable
  Data Store Read3/1 -> GreaterThan/1
